simulink model "FDScanningTool2022b"  (R2022b)
settings: Solver=ode1  StartTime=0.0  StopTime=Tobs  FixedStep=delta_t  RelTol=1e-3
values from neighbouring files (symbols this model uses):
  delta_t = 25E-6    (= 2.5e-05)    [exe_FDScanning.m]    (also in exe_FDScanningTool.m = 1e-05)
  dist_time = dist_time_f    [FDScanning.m]    (also in exe_FDScanningTool.m = 1)
  dist_value_0 = Vsignal_dist3    [FDScanning.m]    (also in exe_FDScanningTool.m = 0.05)
  dist_value_a = [Isignal_dist3(:,1),zeros(samples_window,1)]    [FDScanning.m]    (also in exe_FDScanningTool.m)
  dist_value_b = [Isignal_dist3(:,1),zeros(samples_window,1)]    [FDScanning.m]    (also in exe_FDScanningTool.m)
  dist_value_c = Isignal_dist3    [FDScanning.m]    (also in exe_FDScanningTool.m)
  dist_value_d = Isignal_dist1    [FDScanning.m]    (also in exe_FDScanningTool.m = 0.05)
  dist_value_n = [Vsignal_dist3(:,1),zeros(samples_window,1)]    [FDScanning.m]    (also in exe_FDScanningTool.m = 0)
  dist_value_p = [Vsignal_dist3(:,1),zeros(samples_window,1)]    [FDScanning.m]    (also in exe_FDScanningTool.m = 0)
  dist_value_q = [Isignal_dist1(:,1),zeros(samples_window,1)]    [FDScanning.m]    (also in exe_FDScanningTool.m = 0)
  f0 = fs/Ns    [FDScanning.m]    (also in exe_FDScanning.m = 50; exe_FDScanningTool.m = 50)
  fd = fd0(n)    [FDScanning.m]    (also in exe_FDScanningTool.m)
  Id_ss = 0    [exe_FDScanning.m]
  Ipeak = Sbase/Vpeak    [exe_FDScanning.m]    (also in exe_FDScanningTool.m = 1)
  Iq_ss = 0    [exe_FDScanning.m]
  Iss_type = 2    [FDScanning.m]
  phi = (2/3)*pi    (= 2.09439510239)    [FDScanning.m]    (also in exe_FDScanningTool.m)
  Rsource = 1E-6    (= 1e-06)    [FDScanning.m]    (also in exe_FDScanningTool.m = 0.001)
  signal_type = 3    [exe_FDScanning.m]    (also in exe_FDScanningTool.m = 1)
  Vd_ss = 0    [exe_FDScanning.m]
  Vpeak = (Vbase/sqrt(3))*sqrt(2)    [exe_FDScanning.m]    (also in exe_FDScanningTool.m = 1)
  Vq_ss = 0    [exe_FDScanning.m]
  Vss_type = 2    [FDScanning.m]
libraries: spsControlledCurrentSourceLib x12, spsControlledVoltageSourceLib x12, spsThreePhaseVIMeasurementLib x10, spsGroundLib x2, spsThreePhaseSeriesRLCBranchLib x2, spspowerguiLib x1
(part 1 of 2)
settings Model: SimulationMode=accelerator  Creator=Luis Angel  LastModifiedBy=GARREYLU

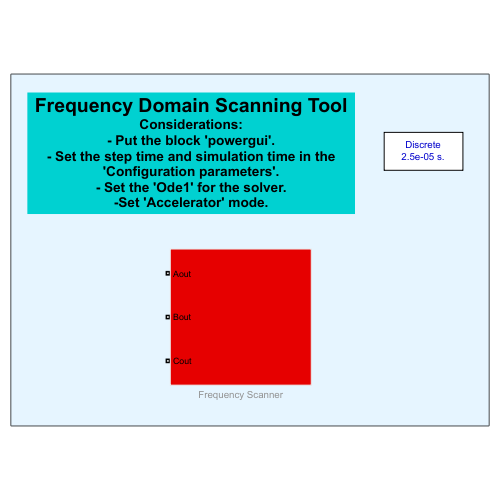
[thumbnail: Simulink's stored preview of the top-level diagram]
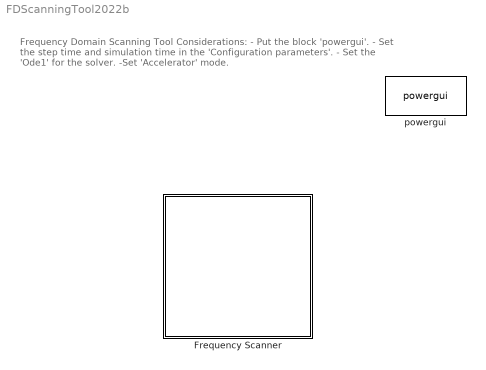
== system FDScanningTool2022b ==
  note: Frequency Domain Scanning Tool
      | Considerations:
      | - Put the block 'powergui'.
      | - Set the step time and simulation time in the 'Configuration parameters'.
      | - Set the 'Ode1' for the solver.
      | -Set 'Accelerator' mode.
  Frequency Scanner : Subsystem
  powergui : spspowerguiLib/powergui  Priority=1  SimulationMode=Discrete  SampleTime=delta_t  frequency=60  Iterations=50  frequencyindice=0  Pbase=100e6  ErrMax=1e-4  UnitsV=kV  UnitsW=MW  buscounter=0  FunctionMessages=off  echomessages=off  EnableUseOfTLC=off  CurrentSourceSwitches=off  DisableSnubberDevices=off  DisableRonSwitches=off  DisableVfSwitches=off  DisplayEquations=off  AutomaticDiscreteSolvers=off  SolverType=Tustin/Backward Euler (TBE)  Interpol=off  ExternalGateDelay=off  methode=off  Ts=100  x0status=blocks  SPID=on  SwTol=0  HookPort=off  NonlinearTolerance=1e-4  nMaxIteration=100  ContinueOnMaxIteration=off  RestoreLinks=warning  ResistiveCurrentMeasurement=off  Frange=[0:2:500]  Ylog=off  Xlog=on  ShowGrid=off  save=off  variable=ZData  structure=0  ZoomFFT=off  StartTime=0.0  cycles=1  DisplayStyle=1  fundamental=60  FreqAxis=off  MaxFrequency=1000  frequencyindicesteady=1  RmsSteady=1  display=off

== system FDScanningTool2022b/Frequency Scanner ==
  note: Current perturbation method
  note: Voltage perturbation method
  Current Strategy : Subsystem  Commented=on
  Three-Phase V-I Measurement1 : spsThreePhaseVIMeasurementLib/Three-Phase V-I Measurement  VoltageMeasurement=no  SetLabelV=on  LabelV=Vabc  Vpu=off  VpuLL=off  CurrentMeasurement=no  SetLabelI=on  LabelI=Iabc  Ipu=off  Pbase=100e6  Vbase=500e3  OutputType=Complex  PhasorSimulation=off  PSBequivalent=0
  Three-Phase V-I Measurement3 : spsThreePhaseVIMeasurementLib/Three-Phase V-I Measurement  VoltageMeasurement=no  SetLabelV=on  LabelV=Vabc  Vpu=off  VpuLL=off  CurrentMeasurement=no  SetLabelI=on  LabelI=Iabc  Ipu=off  Pbase=100e6  Vbase=500e3  OutputType=Complex  PhasorSimulation=off  PSBequivalent=0
  Voltage Strategy : Subsystem
  Aout : PMIOPort  Side=Right
  Bout : PMIOPort  Port=2  Side=Right
  Cout : PMIOPort  Port=3  Side=Right
  connections:
  Bout/RConn1 -- Three-Phase V-I Measurement3/RConn2 -- Three-Phase V-I Measurement1/RConn2
  Aout/RConn1 -- Three-Phase V-I Measurement3/RConn1 -- Three-Phase V-I Measurement1/RConn1
  Cout/RConn1 -- Three-Phase V-I Measurement1/RConn3 -- Three-Phase V-I Measurement3/RConn3
  Three-Phase V-I Measurement1/LConn1 -- Voltage Strategy/RConn1
  Three-Phase V-I Measurement1/LConn2 -- Voltage Strategy/RConn2
  Three-Phase V-I Measurement1/LConn3 -- Voltage Strategy/RConn3
  Three-Phase V-I Measurement3/LConn1 -- Current Strategy/LConn1
  Three-Phase V-I Measurement3/LConn2 -- Current Strategy/LConn2
  Three-Phase V-I Measurement3/LConn3 -- Current Strategy/LConn3

== system FDScanningTool2022b/Frequency Scanner/Current Strategy ==
  note: qd0 scan
  note: Fundamental source
  note: pn0 scan
  note: ABC scan
  ABCdisturbance2 : Subsystem  Commented=on
  Current Fundamental Source : Subsystem
      settings: PortSchema="{\"entries\":[{\"content\":{\"sides\":[{\"content\":{\"connectorIds\":[\"Out1\"]},\"type\":\"ConnectorPlacement.EquallySpacedRectSide\",\"uuid\":\"2a4baa29-0316-4256-b4e1-e3ef1d370b3b\"},{\"content\":{\"connectorIds\":[\"RConn1\",\"RConn2\",\"RConn3\"],\"side\":\"RIGHT\"},\"type\":\"ConnectorPlacement.EquallySpacedRectSide\",\"uuid\":\"3108b85a-ac52-49ed-83a6-d77923640585\"},{\"content\":{\"connectorIds\":[],\"side\":\"TOP\"},\"type\":\"ConnectorPlacement.EquallySpacedRectSide\",\"uuid\":\"4093502e-3b8b-4232-aa57-5a461ca3ca63\"},{\"content\":{\"connectorIds\":[\"RConn4\"],\"side\":\"BOTTOM\"},\"type\":\"ConnectorPlacement.EquallySpacedRectSide\",\"uuid\":\"50c06102-7582-4746-a571-3f791f943454\"}]},\"type\":\"ConnectorPlacement.EquallySpacedConnector\",\"uuid\":\"209f4db4-fe77-48a5-84ae-6773984a343b\"}],\"packageUris\":[\"http://schema.mathworks.com/mf0/Connector/R2020b\"],\"version\":\"1.0\"}"
  Three-Phase V-I Measurement2 : spsThreePhaseVIMeasurementLib/Three-Phase V-I Measurement  VoltageMeasurement=no  SetLabelV=on  LabelV=Vabc  Vpu=off  VpuLL=off  CurrentMeasurement=no  SetLabelI=on  LabelI=Iabc  Ipu=off  Pbase=100e6  Vbase=500e3  OutputType=Complex  PhasorSimulation=off  PSBequivalent=0
  pn0disturbance2 : Subsystem  Commented=on
  qd0disturbance2 : Subsystem
      settings: PortSchema="{\"entries\":[{\"content\":{\"sides\":[{\"content\":{\"connectorIds\":[\"LConn1\",\"LConn2\",\"LConn3\",\"LConn4\"]},\"type\":\"ConnectorPlacement.EquallySpacedRectSide\",\"uuid\":\"96b61a08-e73c-4bf9-b44c-8e6d57b8ef4a\"},{\"content\":{\"connectorIds\":[\"RConn1\",\"RConn2\",\"RConn3\"],\"side\":\"RIGHT\"},\"type\":\"ConnectorPlacement.EquallySpacedRectSide\",\"uuid\":\"3a0e4222-9b60-4a58-9d08-3b159ebff1b9\"},{\"content\":{\"connectorIds\":[\"In1\"],\"side\":\"TOP\"},\"type\":\"ConnectorPlacement.EquallySpacedRectSide\",\"uuid\":\"61af63da-f353-4270-b8c9-89c35459604e\"}]},\"type\":\"ConnectorPlacement.EquallySpacedConnector\",\"uuid\":\"24d596f4-e3d4-42a2-b524-8b1140a91bdb\"}],\"packageUris\":[\"http://schema.mathworks.com/mf0/Connector/R2020b\"],\"version\":\"1.0\"}"
  Aout : PMIOPort  Side=Left
  Bout : PMIOPort  Port=2  Side=Left
  Cout : PMIOPort  Port=3  Side=Left
  wires:
  [theta] -> qd0disturbance2/1(theta)
  Current Fundamental Source/1(theta) -> [theta]
  connections:
  pn0disturbance2/RConn1 -- Aout/RConn1 -- ABCdisturbance2/RConn1 -- qd0disturbance2/RConn1
  pn0disturbance2/RConn2 -- Bout/RConn1 -- ABCdisturbance2/RConn2 -- qd0disturbance2/RConn2
  Current Fundamental Source/RConn2 -- Three-Phase V-I Measurement2/LConn2
  Three-Phase V-I Measurement2/RConn2 -- pn0disturbance2/LConn2 -- ABCdisturbance2/LConn2 -- qd0disturbance2/LConn2
  Current Fundamental Source/RConn3 -- Three-Phase V-I Measurement2/LConn3
  pn0disturbance2/RConn3 -- Cout/RConn1 -- ABCdisturbance2/RConn3 -- qd0disturbance2/RConn3
  Three-Phase V-I Measurement2/RConn1 -- pn0disturbance2/LConn1 -- ABCdisturbance2/LConn1 -- qd0disturbance2/LConn1
  Current Fundamental Source/RConn4 -- pn0disturbance2/LConn4 -- ABCdisturbance2/LConn4 -- qd0disturbance2/LConn4
  Three-Phase V-I Measurement2/RConn3 -- pn0disturbance2/LConn3 -- ABCdisturbance2/LConn3 -- qd0disturbance2/LConn3
  Current Fundamental Source/RConn1 -- Three-Phase V-I Measurement2/LConn1

== system FDScanningTool2022b/Frequency Scanner/Voltage Strategy ==
  note: Fundamental source
  note: pn0 scan
  note: ABC scan
  note: qd0 scan
  ABCdisturbance : Subsystem  Commented=on
  Three-Phase V-I Measurement : spsThreePhaseVIMeasurementLib/Three-Phase V-I Measurement  VoltageMeasurement=no  SetLabelV=on  LabelV=Vabc  Vpu=off  VpuLL=off  CurrentMeasurement=no  SetLabelI=on  LabelI=Iabc  Ipu=off  Pbase=100e6  Vbase=500e3  OutputType=Complex  PhasorSimulation=off  PSBequivalent=0
  Voltage Fundamental Source : Subsystem
      settings: PortSchema="{\"entries\":[{\"content\":{\"sides\":[{\"content\":{\"connectorIds\":[\"Out1\"]},\"type\":\"ConnectorPlacement.EquallySpacedRectSide\",\"uuid\":\"3dbf8d23-22ab-4ddc-ae4a-19197e180312\"},{\"content\":{\"connectorIds\":[\"RConn1\",\"RConn2\",\"RConn3\"],\"side\":\"RIGHT\"},\"type\":\"ConnectorPlacement.EquallySpacedRectSide\",\"uuid\":\"df914263-db35-4888-aa99-5dec7a54c6e0\"},{\"content\":{\"connectorIds\":[],\"side\":\"TOP\"},\"type\":\"ConnectorPlacement.EquallySpacedRectSide\",\"uuid\":\"815bd59d-9d4f-4637-8c0a-95368e7d07f9\"}]},\"type\":\"ConnectorPlacement.EquallySpacedConnector\",\"uuid\":\"b7ffca83-a6f6-4340-8cfa-6aec16cec0d1\"}],\"packageUris\":[\"http://schema.mathworks.com/mf0/Connector/R2020b\"],\"version\":\"1.0\"}"
  pn0disturbance : Subsystem  Commented=on
  qd0disturbance : Subsystem
      settings: PortSchema="{\"entries\":[{\"content\":{\"sides\":[{\"content\":{\"connectorIds\":[\"LConn1\",\"LConn2\",\"LConn3\"]},\"type\":\"ConnectorPlacement.EquallySpacedRectSide\",\"uuid\":\"96b61a08-e73c-4bf9-b44c-8e6d57b8ef4a\"},{\"content\":{\"connectorIds\":[\"RConn1\",\"RConn2\",\"RConn3\"],\"side\":\"RIGHT\"},\"type\":\"ConnectorPlacement.EquallySpacedRectSide\",\"uuid\":\"3a0e4222-9b60-4a58-9d08-3b159ebff1b9\"},{\"content\":{\"connectorIds\":[\"In1\"],\"side\":\"TOP\"},\"type\":\"ConnectorPlacement.EquallySpacedRectSide\",\"uuid\":\"61af63da-f353-4270-b8c9-89c35459604e\"}]},\"type\":\"ConnectorPlacement.EquallySpacedConnector\",\"uuid\":\"24d596f4-e3d4-42a2-b524-8b1140a91bdb\"}],\"packageUris\":[\"http://schema.mathworks.com/mf0/Connector/R2020b\"],\"version\":\"1.0\"}"
  Aout : PMIOPort  Side=Right
  Bout : PMIOPort  Port=2  Side=Right
  Cout : PMIOPort  Port=3  Side=Right
  wires:
  Voltage Fundamental Source/1(theta) -> [theta]
  [theta] -> qd0disturbance/1(theta)
  connections:
  ABCdisturbance/RConn2 -- Bout/RConn1 -- pn0disturbance/RConn2 -- qd0disturbance/RConn2
  Voltage Fundamental Source/RConn1 -- Three-Phase V-I Measurement/LConn1
  qd0disturbance/LConn3 -- ABCdisturbance/LConn3 -- Three-Phase V-I Measurement/RConn3 -- pn0disturbance/LConn3
  ABCdisturbance/RConn1 -- Aout/RConn1 -- pn0disturbance/RConn1 -- qd0disturbance/RConn1
  Voltage Fundamental Source/RConn2 -- Three-Phase V-I Measurement/LConn2
  Voltage Fundamental Source/RConn3 -- Three-Phase V-I Measurement/LConn3
  ABCdisturbance/RConn3 -- Cout/RConn1 -- pn0disturbance/RConn3 -- qd0disturbance/RConn3
  qd0disturbance/LConn1 -- ABCdisturbance/LConn1 -- Three-Phase V-I Measurement/RConn1 -- pn0disturbance/LConn1
  qd0disturbance/LConn2 -- ABCdisturbance/LConn2 -- Three-Phase V-I Measurement/RConn2 -- pn0disturbance/LConn2

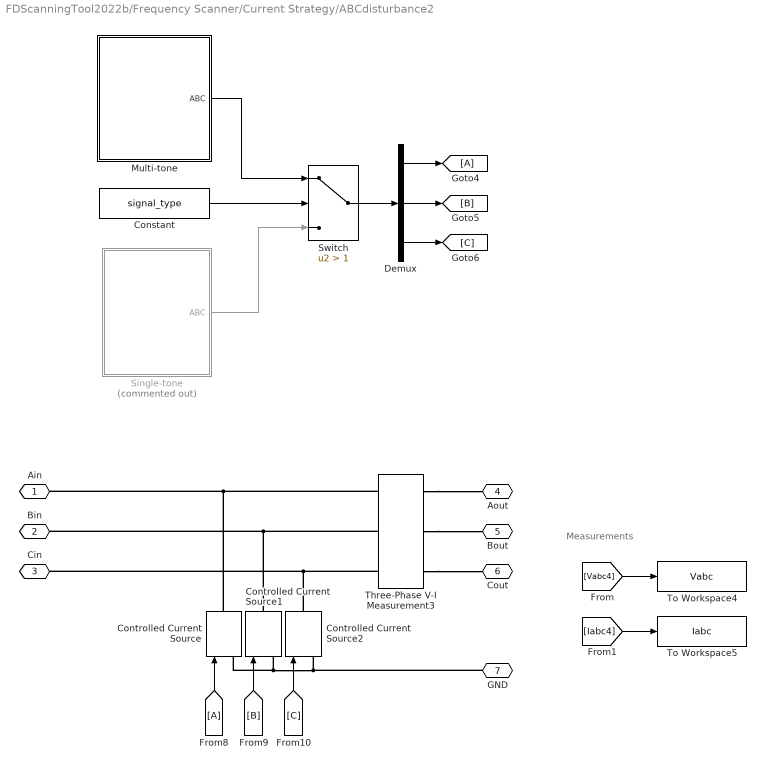
== system FDScanningTool2022b/Frequency Scanner/Current Strategy/ABCdisturbance2 ==
  note: Measurements
  Constant : Constant  Value=signal_type
  Controlled Current Source : spsControlledCurrentSourceLib/Controlled Current Source  Initialize=off  Source_Type=AC  Amplitude=0  Phase=0  Frequency=0  Measurements=None
  Controlled Current Source1 : spsControlledCurrentSourceLib/Controlled Current Source  Initialize=off  Source_Type=AC  Amplitude=0  Phase=0  Frequency=0  Measurements=None
  Controlled Current Source2 : spsControlledCurrentSourceLib/Controlled Current Source  Initialize=off  Source_Type=AC  Amplitude=0  Phase=0  Frequency=0  Measurements=None
  Demux : Demux  Outputs=3
  From8 : From
  Goto4 : Goto
  Multi-tone : Subsystem
  Single-tone : Subsystem  Commented=on
  Switch : Switch  Criteria=u2 > Threshold  Threshold=1  SaturateOnIntegerOverflow=off  InputSameDT=off
  Three-Phase V-I Measurement3 : spsThreePhaseVIMeasurementLib/Three-Phase V-I Measurement  VoltageMeasurement=phase-to-ground  SetLabelV=on  LabelV=Vabc4  Vpu=off  VpuLL=off  CurrentMeasurement=yes  SetLabelI=on  LabelI=Iabc4  Ipu=off  Pbase=100e6  Vbase=500e3  OutputType=Complex  PhasorSimulation=off  PSBequivalent=0
  To Workspace4 : ToWorkspace  VariableName=Vabc  SampleTime=-1
  To Workspace5 : ToWorkspace  VariableName=Iabc  SampleTime=-1
  Ain : PMIOPort  Side=Left
  Bin : PMIOPort  Port=2  Side=Left
  Cin : PMIOPort  Port=3  Side=Left
  Aout : PMIOPort  Port=4  Side=Right
  Bout : PMIOPort  Port=5  Side=Right
  Cout : PMIOPort  Port=6  Side=Right
  GND : PMIOPort  Port=7  Side=Left
  wires:
  [Vabc4] -> To Workspace4/1
  [Iabc4] -> To Workspace5/1
  [C] -> Controlled Current Source2/1
  [B] -> Controlled Current Source1/1
  From8/1 -> Controlled Current Source/1
  Constant/1 -> Switch/2
  Multi-tone/1(ABC) -> Switch/1
  Demux/1 -> Goto4/1
  Demux/2 -> [B]
  Demux/3 -> [C]
  Switch/1 -> Demux/1
  Single-tone/1(ABC) -> Switch/3
  connections:
  Controlled Current Source1/LConn1 -- GND/RConn1 -- Controlled Current Source2/LConn1 -- Controlled Current Source/LConn1
  Controlled Current Source/RConn1 -- Three-Phase V-I Measurement3/LConn1 -- Ain/RConn1
  Controlled Current Source2/RConn1 -- Three-Phase V-I Measurement3/LConn3 -- Cin/RConn1
  Controlled Current Source1/RConn1 -- Three-Phase V-I Measurement3/LConn2 -- Bin/RConn1
  Three-Phase V-I Measurement3/RConn1 -- Aout/RConn1
  Three-Phase V-I Measurement3/RConn2 -- Bout/RConn1
  Three-Phase V-I Measurement3/RConn3 -- Cout/RConn1

== system FDScanningTool2022b/Frequency Scanner/Current Strategy/Current Fundamental Source ==
  Controlled Current Source : spsControlledCurrentSourceLib/Controlled Current Source  Initialize=off  Source_Type=AC  Amplitude=0  Phase=0  Frequency=0  Measurements=None
  Controlled Current Source1 : spsControlledCurrentSourceLib/Controlled Current Source  Initialize=off  Source_Type=AC  Amplitude=0  Phase=0  Frequency=0  Measurements=None
  Controlled Current Source2 : spsControlledCurrentSourceLib/Controlled Current Source  Initialize=off  Source_Type=AC  Amplitude=0  Phase=0  Frequency=0  Measurements=None
  Grid Currents1 : Subsystem
  Ground : spsGroundLib/Ground  LConnTagsString=a
  Three-Phase Series RLC Branch : spsThreePhaseSeriesRLCBranchLib/Three-Phase Series RLC Branch  LConnTagsString=A|B|C  RConnTagsString=A|B|C  BranchType=R  Resistance=1/Rsource  Inductance=1e-3  Capacitance=1e-6  Measurements=None
  VzA : PMIOPort  Side=Right
  VzB : PMIOPort  Port=2  Side=Right
  VzC : PMIOPort  Port=3  Side=Right
  GND : PMIOPort  Port=4  Side=Right
  theta : Outport
  wires:
  Grid Currents1/3(IC) -> Controlled Current Source/1
  Grid Currents1/2(IB) -> Controlled Current Source1/1
  Grid Currents1/1(IA) -> Controlled Current Source2/1
  Grid Currents1/4(theta) -> theta/1
  connections:
  Controlled Current Source2/RConn1 -- Three-Phase Series RLC Branch/LConn1 -- VzA/RConn1
  Controlled Current Source1/RConn1 -- Three-Phase Series RLC Branch/LConn2 -- VzB/RConn1
  Controlled Current Source/RConn1 -- Three-Phase Series RLC Branch/LConn3 -- VzC/RConn1
  Ground/LConn1 -- Controlled Current Source/LConn1 -- Controlled Current Source1/LConn1 -- Controlled Current Source2/LConn1 -- Three-Phase Series RLC Branch/RConn3 -- Three-Phase Series RLC Branch/RConn2 -- Three-Phase Series RLC Branch/RConn1 -- GND/RConn1

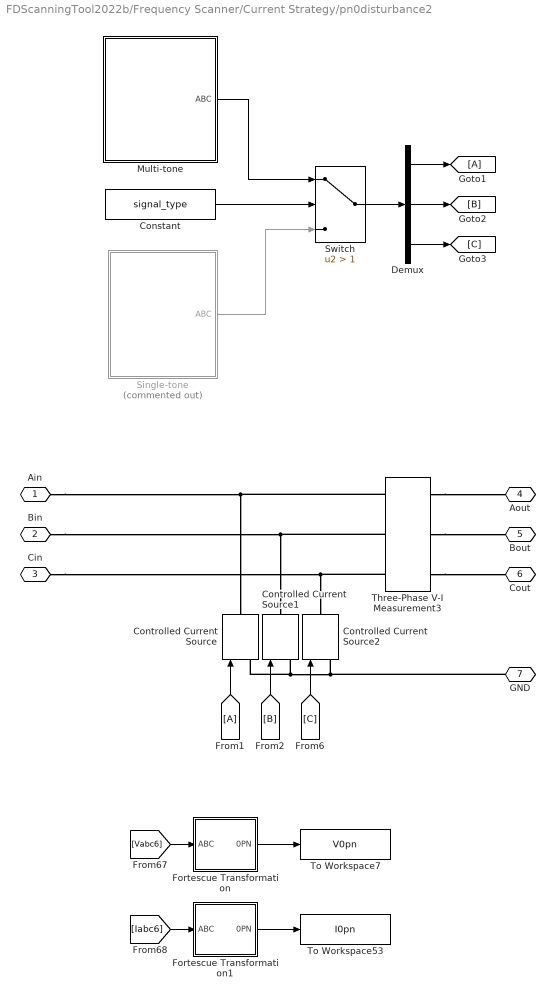
== system FDScanningTool2022b/Frequency Scanner/Current Strategy/pn0disturbance2 ==
  Constant : Constant  Value=signal_type
  Controlled Current Source : spsControlledCurrentSourceLib/Controlled Current Source  Initialize=off  Source_Type=AC  Amplitude=0  Phase=0  Frequency=0  Measurements=None
  Controlled Current Source1 : spsControlledCurrentSourceLib/Controlled Current Source  Initialize=off  Source_Type=AC  Amplitude=0  Phase=0  Frequency=0  Measurements=None
  Controlled Current Source2 : spsControlledCurrentSourceLib/Controlled Current Source  Initialize=off  Source_Type=AC  Amplitude=0  Phase=0  Frequency=0  Measurements=None
  Demux : Demux  Outputs=3
  Fortescue Transformation : Subsystem
  Fortescue Transformation1 : Subsystem
  From1 : From
  Goto1 : Goto
  Multi-tone : Subsystem
  Single-tone : Subsystem  Commented=on
  Switch : Switch  Criteria=u2 > Threshold  Threshold=1  SaturateOnIntegerOverflow=off  InputSameDT=off
  Three-Phase V-I Measurement3 : spsThreePhaseVIMeasurementLib/Three-Phase V-I Measurement  VoltageMeasurement=phase-to-ground  SetLabelV=on  LabelV=Vabc6  Vpu=off  VpuLL=off  CurrentMeasurement=yes  SetLabelI=on  LabelI=Iabc6  Ipu=off  Pbase=100e6  Vbase=500e3  OutputType=Complex  PhasorSimulation=off  PSBequivalent=0
  To Workspace53 : ToWorkspace  VariableName=I0pn  SampleTime=-1
  To Workspace7 : ToWorkspace  VariableName=V0pn  SampleTime=-1
  Ain : PMIOPort  Side=Left
  Bin : PMIOPort  Port=2  Side=Left
  Cin : PMIOPort  Port=3  Side=Left
  Aout : PMIOPort  Port=4  Side=Right
  Bout : PMIOPort  Port=5  Side=Right
  Cout : PMIOPort  Port=6  Side=Right
  GND : PMIOPort  Port=7  Side=Left
  wires:
  [Vabc6] -> Fortescue Transformation/1(ABC)
  [Iabc6] -> Fortescue Transformation1/1(ABC)
  Fortescue Transformation/1(0PN) -> To Workspace7/1
  Fortescue Transformation1/1(0PN) -> To Workspace53/1
  [B] -> Controlled Current Source1/1
  [C] -> Controlled Current Source2/1
  From1/1 -> Controlled Current Source/1
  Multi-tone/1(ABC) -> Switch/1
  Demux/1 -> Goto1/1
  Demux/3 -> [C]
  Constant/1 -> Switch/2
  Single-tone/1(ABC) -> Switch/3
  Switch/1 -> Demux/1
  Demux/2 -> [B]
  connections:
  Cin/RConn1 -- Three-Phase V-I Measurement3/LConn3 -- Controlled Current Source2/RConn1
  Controlled Current Source1/LConn1 -- GND/RConn1 -- Controlled Current Source2/LConn1 -- Controlled Current Source/LConn1
  Ain/RConn1 -- Three-Phase V-I Measurement3/LConn1 -- Controlled Current Source/RConn1
  Bin/RConn1 -- Three-Phase V-I Measurement3/LConn2 -- Controlled Current Source1/RConn1
  Three-Phase V-I Measurement3/RConn3 -- Cout/RConn1
  Three-Phase V-I Measurement3/RConn2 -- Bout/RConn1
  Three-Phase V-I Measurement3/RConn1 -- Aout/RConn1

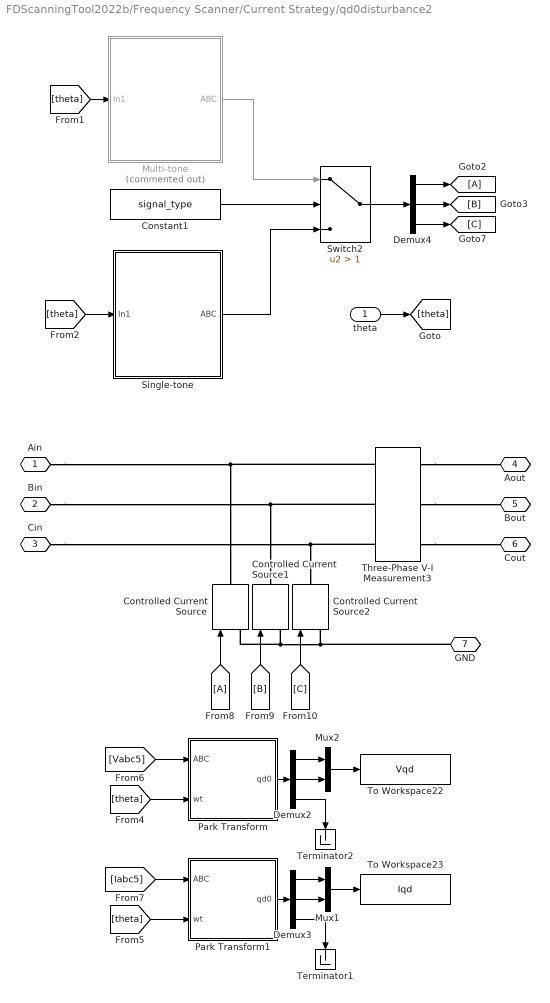
== system FDScanningTool2022b/Frequency Scanner/Current Strategy/qd0disturbance2 ==
  theta : Inport
  Constant1 : Constant  Value=signal_type
  Controlled Current Source : spsControlledCurrentSourceLib/Controlled Current Source  Initialize=off  Source_Type=AC  Amplitude=0  Phase=0  Frequency=0  Measurements=None
  Controlled Current Source1 : spsControlledCurrentSourceLib/Controlled Current Source  Initialize=off  Source_Type=AC  Amplitude=0  Phase=0  Frequency=0  Measurements=None
  Controlled Current Source2 : spsControlledCurrentSourceLib/Controlled Current Source  Initialize=off  Source_Type=AC  Amplitude=0  Phase=0  Frequency=0  Measurements=None
  Demux2 : Demux  Outputs=3
  Demux3 : Demux  Outputs=3
  Demux4 : Demux  Outputs=3
  From8 : From
  Goto2 : Goto
  Multi-tone : Subsystem  Commented=on
  Mux1 : Mux  Inputs=2
  Mux2 : Mux  Inputs=2
  Park Transform : Subsystem
  Park Transform1 : Subsystem
  Single-tone : Subsystem
  Switch2 : Switch  Criteria=u2 > Threshold  Threshold=1  SaturateOnIntegerOverflow=off  InputSameDT=off
  Terminator1 : Terminator
  Terminator2 : Terminator
  Three-Phase V-I Measurement3 : spsThreePhaseVIMeasurementLib/Three-Phase V-I Measurement  VoltageMeasurement=phase-to-ground  SetLabelV=on  LabelV=Vabc5  Vpu=off  VpuLL=off  CurrentMeasurement=yes  SetLabelI=on  LabelI=Iabc5  Ipu=off  Pbase=100e6  Vbase=500e3  OutputType=Complex  PhasorSimulation=off  PSBequivalent=0
  To Workspace22 : ToWorkspace  VariableName=Vqd  SampleTime=-1
  To Workspace23 : ToWorkspace  VariableName=Iqd  SampleTime=-1
  Ain : PMIOPort  Side=Left
  Bin : PMIOPort  Port=2  Side=Left
  Cin : PMIOPort  Port=3  Side=Left
  Aout : PMIOPort  Port=4  Side=Right
  Bout : PMIOPort  Port=5  Side=Right
  Cout : PMIOPort  Port=6  Side=Right
  GND : PMIOPort  Port=7  Side=Left
  wires:
  Mux2/1 -> To Workspace22/1
  [theta] -> Park Transform/2(wt)
  [Vabc5] -> Park Transform/1(ABC)
  Park Transform/1(qd0) -> Demux2/1
  Demux2/3 -> Terminator2/1
  theta/1 -> [theta]
  Demux2/1 -> Mux2/1
  Demux2/2 -> Mux2/2
  Mux1/1 -> To Workspace23/1
  Demux3/3 -> Terminator1/1
  [Iabc5] -> Park Transform1/1(ABC)
  Park Transform1/1(qd0) -> Demux3/1
  Demux3/2 -> Mux1/2
  Demux3/1 -> Mux1/1
  [theta] -> Park Transform1/2(wt)
  From8/1 -> Controlled Current Source/1
  [C] -> Controlled Current Source2/1
  [B] -> Controlled Current Source1/1
  Constant1/1 -> Switch2/2
  Multi-tone/1(ABC) -> Switch2/1
  [theta] -> Single-tone/1(In1)
  Switch2/1 -> Demux4/1
  Single-tone/1(ABC) -> Switch2/3
  Demux4/1 -> Goto2/1
  Demux4/2 -> [B]
  [theta] -> Multi-tone/1(In1)
  Demux4/3 -> [C]
  connections:
  Controlled Current Source1/LConn1 -- GND/RConn1 -- Controlled Current Source2/LConn1 -- Controlled Current Source/LConn1
  Ain/RConn1 -- Three-Phase V-I Measurement3/LConn1 -- Controlled Current Source/RConn1
  Bin/RConn1 -- Three-Phase V-I Measurement3/LConn2 -- Controlled Current Source1/RConn1
  Cin/RConn1 -- Three-Phase V-I Measurement3/LConn3 -- Controlled Current Source2/RConn1
  Three-Phase V-I Measurement3/RConn1 -- Aout/RConn1
  Three-Phase V-I Measurement3/RConn2 -- Bout/RConn1
  Three-Phase V-I Measurement3/RConn3 -- Cout/RConn1

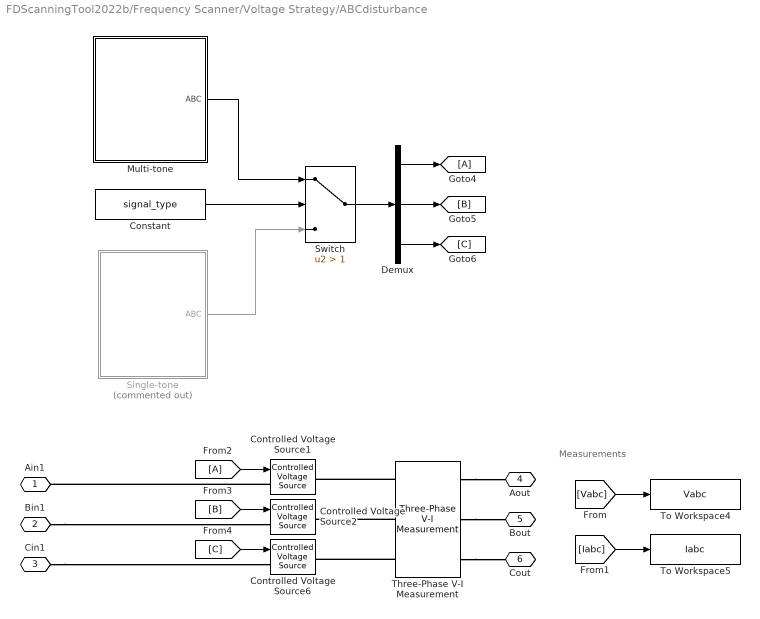
== system FDScanningTool2022b/Frequency Scanner/Voltage Strategy/ABCdisturbance ==
  note: Measurements
  Constant : Constant  Value=signal_type
  Controlled Voltage Source1 : spsControlledVoltageSourceLib/Controlled Voltage Source  Initialize=off  Source_Type=DC  Amplitude=0  Phase=0  Frequency=0  Measurements=None
  Controlled Voltage Source2 : spsControlledVoltageSourceLib/Controlled Voltage Source  Initialize=off  Source_Type=DC  Amplitude=0  Phase=0  Frequency=0  Measurements=None
  Controlled Voltage Source6 : spsControlledVoltageSourceLib/Controlled Voltage Source  Initialize=off  Source_Type=DC  Amplitude=0  Phase=0  Frequency=0  Measurements=None
  Demux : Demux  Outputs=3
  From2 : From
  Goto4 : Goto
  Multi-tone : Subsystem
  Single-tone : Subsystem  Commented=on
  Switch : Switch  Criteria=u2 > Threshold  Threshold=1  SaturateOnIntegerOverflow=off  InputSameDT=off
  Three-Phase V-I Measurement : spsThreePhaseVIMeasurementLib/Three-Phase V-I Measurement  VoltageMeasurement=phase-to-ground  SetLabelV=on  LabelV=Vabc  Vpu=off  VpuLL=off  CurrentMeasurement=yes  SetLabelI=on  LabelI=Iabc  Ipu=off  Pbase=100e6  Vbase=500e3  OutputType=Complex  PhasorSimulation=off  PSBequivalent=0
  To Workspace4 : ToWorkspace  VariableName=Vabc  SampleTime=-1
  To Workspace5 : ToWorkspace  VariableName=Iabc  SampleTime=-1
  Ain1 : PMIOPort  Side=Left
  Bin1 : PMIOPort  Port=2  Side=Left
  Cin1 : PMIOPort  Port=3  Side=Left
  Aout : PMIOPort  Port=4  Side=Right
  Bout : PMIOPort  Port=5  Side=Right
  Cout : PMIOPort  Port=6  Side=Right
  wires:
  [Vabc] -> To Workspace4/1
  [Iabc] -> To Workspace5/1
  [C] -> Controlled Voltage Source6/1
  From2/1 -> Controlled Voltage Source1/1
  [B] -> Controlled Voltage Source2/1
  Multi-tone/1(ABC) -> Switch/1
  Demux/3 -> [C]
  Constant/1 -> Switch/2
  Demux/1 -> Goto4/1
  Demux/2 -> [B]
  Single-tone/1(ABC) -> Switch/3
  Switch/1 -> Demux/1
  connections:
  Bin1/RConn1 -- Controlled Voltage Source2/LConn1
  Controlled Voltage Source1/LConn1 -- Ain1/RConn1
  Cin1/RConn1 -- Controlled Voltage Source6/LConn1
  Three-Phase V-I Measurement/LConn1 -- Controlled Voltage Source1/RConn1
  Three-Phase V-I Measurement/LConn2 -- Controlled Voltage Source2/RConn1
  Three-Phase V-I Measurement/LConn3 -- Controlled Voltage Source6/RConn1
  Three-Phase V-I Measurement/RConn3 -- Cout/RConn1
  Three-Phase V-I Measurement/RConn2 -- Bout/RConn1
  Three-Phase V-I Measurement/RConn1 -- Aout/RConn1

== system FDScanningTool2022b/Frequency Scanner/Voltage Strategy/Voltage Fundamental Source ==
  Controlled Voltage Source1 : spsControlledVoltageSourceLib/Controlled Voltage Source  Initialize=off  Source_Type=DC  Amplitude=0  Phase=0  Frequency=0  Measurements=None
  Controlled Voltage Source2 : spsControlledVoltageSourceLib/Controlled Voltage Source  Initialize=off  Source_Type=DC  Amplitude=0  Phase=0  Frequency=0  Measurements=None
  Controlled Voltage Source3 : spsControlledVoltageSourceLib/Controlled Voltage Source  Initialize=off  Source_Type=DC  Amplitude=0  Phase=0  Frequency=0  Measurements=None
  Grid Voltages : Subsystem
  Ground : spsGroundLib/Ground  LConnTagsString=a
  Three-Phase Series RLC Branch : spsThreePhaseSeriesRLCBranchLib/Three-Phase Series RLC Branch  LConnTagsString=A|B|C  RConnTagsString=A|B|C  BranchType=R  Resistance=Rsource  Inductance=1e-3  Capacitance=1e-6  Measurements=None
  VzA : PMIOPort  Side=Right
  VzB : PMIOPort  Port=2  Side=Right
  VzC : PMIOPort  Port=3  Side=Right
  theta : Outport
  wires:
  Grid Voltages/3(VC) -> Controlled Voltage Source3/1
  Grid Voltages/2(VB) -> Controlled Voltage Source2/1
  Grid Voltages/1(VA) -> Controlled Voltage Source1/1
  Grid Voltages/4(theta) -> theta/1
  connections:
  Controlled Voltage Source2/LConn1 -- Controlled Voltage Source1/LConn1 -- Controlled Voltage Source3/LConn1 -- Ground/LConn1
  Three-Phase Series RLC Branch/RConn1 -- Controlled Voltage Source1/RConn1
  Three-Phase Series RLC Branch/RConn2 -- Controlled Voltage Source2/RConn1
  Three-Phase Series RLC Branch/RConn3 -- Controlled Voltage Source3/RConn1
  Three-Phase Series RLC Branch/LConn3 -- VzC/RConn1
  Three-Phase Series RLC Branch/LConn2 -- VzB/RConn1
  Three-Phase Series RLC Branch/LConn1 -- VzA/RConn1

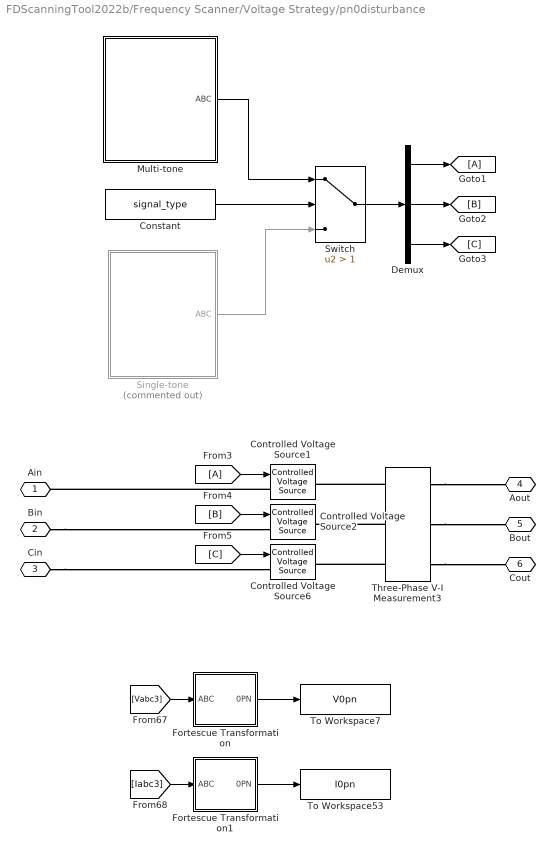
== system FDScanningTool2022b/Frequency Scanner/Voltage Strategy/pn0disturbance ==
  Constant : Constant  Value=signal_type
  Controlled Voltage Source1 : spsControlledVoltageSourceLib/Controlled Voltage Source  Initialize=off  Source_Type=DC  Amplitude=0  Phase=0  Frequency=0  Measurements=None
  Controlled Voltage Source2 : spsControlledVoltageSourceLib/Controlled Voltage Source  Initialize=off  Source_Type=DC  Amplitude=0  Phase=0  Frequency=0  Measurements=None
  Controlled Voltage Source6 : spsControlledVoltageSourceLib/Controlled Voltage Source  Initialize=off  Source_Type=DC  Amplitude=0  Phase=0  Frequency=0  Measurements=None
  Demux : Demux  Outputs=3
  Fortescue Transformation : Subsystem
  Fortescue Transformation1 : Subsystem
  From3 : From
  Goto1 : Goto
  Multi-tone : Subsystem
  Single-tone : Subsystem  Commented=on
  Switch : Switch  Criteria=u2 > Threshold  Threshold=1  SaturateOnIntegerOverflow=off  InputSameDT=off
  Three-Phase V-I Measurement3 : spsThreePhaseVIMeasurementLib/Three-Phase V-I Measurement  VoltageMeasurement=phase-to-ground  SetLabelV=on  LabelV=Vabc3  Vpu=off  VpuLL=off  CurrentMeasurement=yes  SetLabelI=on  LabelI=Iabc3  Ipu=off  Pbase=100e6  Vbase=500e3  OutputType=Complex  PhasorSimulation=off  PSBequivalent=0
  To Workspace53 : ToWorkspace  VariableName=I0pn  SampleTime=-1
  To Workspace7 : ToWorkspace  VariableName=V0pn  SampleTime=-1
  Ain : PMIOPort  Side=Left
  Bin : PMIOPort  Port=2  Side=Left
  Cin : PMIOPort  Port=3  Side=Left
  Aout : PMIOPort  Port=4  Side=Right
  Bout : PMIOPort  Port=5  Side=Right
  Cout : PMIOPort  Port=6  Side=Right
  wires:
  [B] -> Controlled Voltage Source2/1
  From3/1 -> Controlled Voltage Source1/1
  [C] -> Controlled Voltage Source6/1
  [Vabc3] -> Fortescue Transformation/1(ABC)
  [Iabc3] -> Fortescue Transformation1/1(ABC)
  Fortescue Transformation/1(0PN) -> To Workspace7/1
  Fortescue Transformation1/1(0PN) -> To Workspace53/1
  Switch/1 -> Demux/1
  Single-tone/1(ABC) -> Switch/3
  Demux/3 -> [C]
  Multi-tone/1(ABC) -> Switch/1
  Demux/1 -> Goto1/1
  Demux/2 -> [B]
  Constant/1 -> Switch/2
  connections:
  Controlled Voltage Source1/LConn1 -- Ain/RConn1
  Cin/RConn1 -- Controlled Voltage Source6/LConn1
  Bin/RConn1 -- Controlled Voltage Source2/LConn1
  Three-Phase V-I Measurement3/LConn1 -- Controlled Voltage Source1/RConn1
  Three-Phase V-I Measurement3/LConn2 -- Controlled Voltage Source2/RConn1
  Three-Phase V-I Measurement3/LConn3 -- Controlled Voltage Source6/RConn1
  Three-Phase V-I Measurement3/RConn1 -- Aout/RConn1
  Three-Phase V-I Measurement3/RConn2 -- Bout/RConn1
  Three-Phase V-I Measurement3/RConn3 -- Cout/RConn1

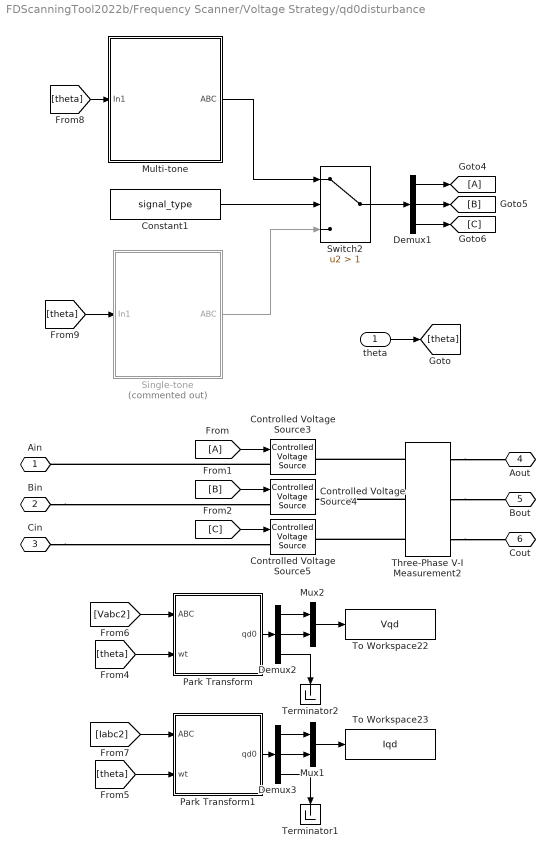
== system FDScanningTool2022b/Frequency Scanner/Voltage Strategy/qd0disturbance ==
  theta : Inport
  Constant1 : Constant  Value=signal_type
  Controlled Voltage Source3 : spsControlledVoltageSourceLib/Controlled Voltage Source  Initialize=off  Source_Type=DC  Amplitude=0  Phase=0  Frequency=0  Measurements=None
  Controlled Voltage Source4 : spsControlledVoltageSourceLib/Controlled Voltage Source  Initialize=off  Source_Type=DC  Amplitude=0  Phase=0  Frequency=0  Measurements=None
  Controlled Voltage Source5 : spsControlledVoltageSourceLib/Controlled Voltage Source  Initialize=off  Source_Type=DC  Amplitude=0  Phase=0  Frequency=0  Measurements=None
  Demux1 : Demux  Outputs=3
  Demux2 : Demux  Outputs=3
  Demux3 : Demux  Outputs=3
  From : From
  Goto4 : Goto
  Multi-tone : Subsystem
  Mux1 : Mux  Inputs=2
  Mux2 : Mux  Inputs=2
  Park Transform : Subsystem
  Park Transform1 : Subsystem
  Single-tone : Subsystem  Commented=on
  Switch2 : Switch  Criteria=u2 > Threshold  Threshold=1  SaturateOnIntegerOverflow=off  InputSameDT=off
  Terminator1 : Terminator
  Terminator2 : Terminator
  Three-Phase V-I Measurement2 : spsThreePhaseVIMeasurementLib/Three-Phase V-I Measurement  VoltageMeasurement=phase-to-ground  SetLabelV=on  LabelV=Vabc2  Vpu=off  VpuLL=off  CurrentMeasurement=yes  SetLabelI=on  LabelI=Iabc2  Ipu=off  Pbase=100e6  Vbase=500e3  OutputType=Complex  PhasorSimulation=off  PSBequivalent=0
  To Workspace22 : ToWorkspace  VariableName=Vqd  SampleTime=-1
  To Workspace23 : ToWorkspace  VariableName=Iqd  SampleTime=-1
  Ain : PMIOPort  Side=Left
  Bin : PMIOPort  Port=2  Side=Left
  Cin : PMIOPort  Port=3  Side=Left
  Aout : PMIOPort  Port=4  Side=Right
  Bout : PMIOPort  Port=5  Side=Right
  Cout : PMIOPort  Port=6  Side=Right
  wires:
  From/1 -> Controlled Voltage Source3/1
  [B] -> Controlled Voltage Source4/1
  [C] -> Controlled Voltage Source5/1
  Mux2/1 -> To Workspace22/1
  [theta] -> Park Transform/2(wt)
  [Vabc2] -> Park Transform/1(ABC)
  Park Transform/1(qd0) -> Demux2/1
  Demux2/3 -> Terminator2/1
  theta/1 -> [theta]
  Demux2/1 -> Mux2/1
  Demux2/2 -> Mux2/2
  Mux1/1 -> To Workspace23/1
  Demux3/3 -> Terminator1/1
  [Iabc2] -> Park Transform1/1(ABC)
  Park Transform1/1(qd0) -> Demux3/1
  Demux3/2 -> Mux1/2
  Demux3/1 -> Mux1/1
  [theta] -> Park Transform1/2(wt)
  Switch2/1 -> Demux1/1
  Single-tone/1(ABC) -> Switch2/3
  Multi-tone/1(ABC) -> Switch2/1
  Constant1/1 -> Switch2/2
  [theta] -> Single-tone/1(In1)
  Demux1/3 -> [C]
  Demux1/1 -> Goto4/1
  Demux1/2 -> [B]
  [theta] -> Multi-tone/1(In1)
  connections:
  Controlled Voltage Source3/LConn1 -- Ain/RConn1
  Bin/RConn1 -- Controlled Voltage Source4/LConn1
  Cin/RConn1 -- Controlled Voltage Source5/LConn1
  Three-Phase V-I Measurement2/LConn1 -- Controlled Voltage Source3/RConn1
  Three-Phase V-I Measurement2/LConn2 -- Controlled Voltage Source4/RConn1
  Three-Phase V-I Measurement2/LConn3 -- Controlled Voltage Source5/RConn1
  Three-Phase V-I Measurement2/RConn1 -- Aout/RConn1
  Three-Phase V-I Measurement2/RConn2 -- Bout/RConn1
  Three-Phase V-I Measurement2/RConn3 -- Cout/RConn1

== system FDScanningTool2022b/Frequency Scanner/Current Strategy/ABCdisturbance2/Multi-tone ==
  Clock : Clock
  Constant1 : Constant  Value=0
  From Workspace : FromWorkspace  VariableName=dist_value_a  SampleTime=delta_t  Interpolate=off  OutputAfterFinalValue=Holding final value
  From Workspace1 : FromWorkspace  VariableName=dist_value_b  SampleTime=delta_t  Interpolate=off  OutputAfterFinalValue=Holding final value
  From Workspace2 : FromWorkspace  VariableName=dist_value_c  SampleTime=delta_t  Interpolate=off  OutputAfterFinalValue=Holding final value
  Mux : Mux  Inputs=3
  Switch1 : Switch  Criteria=u2 > Threshold  Threshold=dist_time  SaturateOnIntegerOverflow=off  InputSameDT=off
  Switch2 : Switch  Criteria=u2 > Threshold  Threshold=dist_time  SaturateOnIntegerOverflow=off  InputSameDT=off
  Switch3 : Switch  Criteria=u2 > Threshold  Threshold=dist_time  SaturateOnIntegerOverflow=off  InputSameDT=off
  ABC : Outport
  wires:
  Switch2/1 -> Mux/2
  From Workspace2/1 -> Switch3/1
  Constant1/1 -> Switch3/3, Switch2/3, Switch1/3
  From Workspace1/1 -> Switch2/1
  Switch3/1 -> Mux/3
  Clock/1 -> Switch1/2, Switch2/2, Switch3/2
  Switch1/1 -> Mux/1
  From Workspace/1 -> Switch1/1
  Mux/1 -> ABC/1

== system FDScanningTool2022b/Frequency Scanner/Current Strategy/ABCdisturbance2/Single-tone ==
  note: ABC perturbance
  Constant10 : Constant  Value=phi
  Constant12 : Constant  Value=2*pi*fd  SampleTime=delta_t
  Constant9 : Constant  Value=phi
  Integrator5 : Integrator  UpperSaturationLimit=1E100  LowerSaturationLimit=-1E100
  Mux : Mux  Inputs=3
  Product1 : Product
  Product2 : Product
  Product3 : Product
  Sin : Trigonometry  Operator=cos
  Sin1 : Trigonometry  Operator=cos
  Sin2 : Trigonometry  Operator=cos
  Step1 : Step  Time=dist_time  After=dist_value_a  SampleTime=delta_t
  Step2 : Step  Time=dist_time  After=dist_value_b  SampleTime=delta_t
  Step3 : Step  Time=dist_time  After=dist_value_c  SampleTime=delta_t
  Sum6 : Sum  Inputs=|+-
  Sum7 : Sum  Inputs=|++
  ABC : Outport
  wires:
  Sin/1 -> Product1/1
  Sum7/1 -> Sin2/1
  Product1/1 -> Mux/1
  Integrator5/1 -> Sum7/1, Sin/1, Sum6/1
  Sin1/1 -> Product2/1
  Sin2/1 -> Product3/1
  Constant9/1 -> Sum6/2
  Constant10/1 -> Sum7/2
  Step3/1 -> Product3/2
  Step2/1 -> Product2/2
  Constant12/1 -> Integrator5/1
  Sum6/1 -> Sin1/1
  Step1/1 -> Product1/2
  Product2/1 -> Mux/2
  Product3/1 -> Mux/3
  Mux/1 -> ABC/1

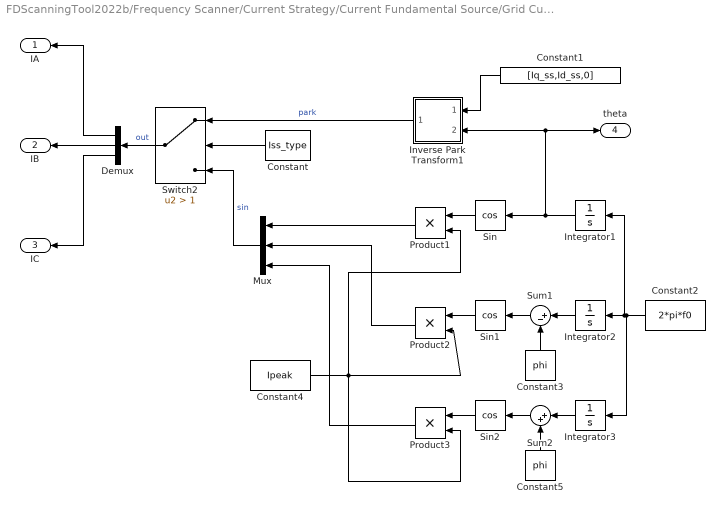
== system FDScanningTool2022b/Frequency Scanner/Current Strategy/Current Fundamental Source/Grid Currents1 ==
  Constant : Constant  Value=Iss_type
  Constant1 : Constant  Value=[Iq_ss,Id_ss,0]  SampleTime=delta_t
  Constant2 : Constant  Value=2*pi*f0
  Constant3 : Constant  Value=phi
  Constant4 : Constant  Value=Ipeak
  Constant5 : Constant  Value=phi
  Demux : Demux  Outputs=3
  Integrator1 : Integrator  UpperSaturationLimit=1E100  LowerSaturationLimit=-1E100
  Integrator2 : Integrator  UpperSaturationLimit=1E100  LowerSaturationLimit=-1E100
  Integrator3 : Integrator  UpperSaturationLimit=1E100  LowerSaturationLimit=-1E100
  Inverse Park Transform1 : Subsystem
  Mux : Mux  Inputs=3
  Product1 : Product
  Product2 : Product
  Product3 : Product
  Sin : Trigonometry  Operator=cos
  Sin1 : Trigonometry  Operator=cos
  Sin2 : Trigonometry  Operator=cos
  Sum1 : Sum  Inputs=|+-
  Sum2 : Sum  Inputs=|++
  Switch2 : Switch  Criteria=u2 > Threshold  Threshold=1  SaturateOnIntegerOverflow=off  InputSameDT=off
  IA : Outport
  IB : Outport  Port=2
  IC : Outport  Port=3
  theta : Outport  Port=4
  wires:
  Constant1/1 -> Inverse Park Transform1/1(qd0)
  Demux/1 -> IA/1
  Demux/2 -> IB/1
  Demux/3 -> IC/1
  Product3/1 -> Mux/3
  Product1/1 -> Mux/1
  Sum1/1 -> Sin1/1
  Integrator2/1 -> Sum1/1
  Constant5/1 -> Sum2/2
  Integrator3/1 -> Sum2/1
  Sin/1 -> Product1/1
  Sin2/1 -> Product3/1
  Sin1/1 -> Product2/1
  Sum2/1 -> Sin2/1
  Constant2/1 -> Integrator1/1, Integrator2/1, Integrator3/1
  Integrator1/1 -> theta/1, Inverse Park Transform1/2(theta), Sin/1
  Constant4/1 -> Product2/2, Product1/2, Product3/2
  Product2/1 -> Mux/2
  Constant3/1 -> Sum1/2
  Switch2/1 -> Demux/1  "out"
  Inverse Park Transform1/1(ABC) -> Switch2/1  "park"
  Mux/1 -> Switch2/3  "sin"
  Constant/1 -> Switch2/2

== system FDScanningTool2022b/Frequency Scanner/Current Strategy/pn0disturbance2/Fortescue Transformation ==
  note: This block buid a column vector with the inputs
      | M=[In1 In2 In3
      |       In1 In2 In3
      |       In1 In2 In3];
  ABC : Inport
  Constant{,3,46..47} (4 alike) : Constant  Value=0
  Constant1 : Constant  Value=(2/3)*pi
  Constant2 : Constant
  Constant43 : Constant
  Constant45 : Constant
  Math Function : Math
  Math Function1 : Math
  Matrix Concatenate : Concatenate  NumInputs=3  Mode=Multidimensional array  ConcatenateDimension=2
  Matrix Multiply : Product  Multiplication=Matrix(*)
  Multiply : Gain  Gain=1/3
  Mux1 : Mux  Inputs=3
  Mux2 : Mux  Inputs=3
  Mux3 : Mux  Inputs=3
  Real-Imag to Complex{,1..2,5} (4 alike) : RealImagToComplex
  Square : Math  Operator=square
  Square1 : Math  Operator=square
  0PN : Outport
  wires:
  Square/1 -> Mux1/3
  Math Function/1 -> Mux1/2, Square/1
  Real-Imag to Complex1/1 -> Mux3/1
  Square1/1 -> Mux3/2
  Multiply/1 -> Matrix Multiply/1
  Math Function1/1 -> Square1/1, Mux3/3
  Mux3/1 -> Matrix Concatenate/3
  Constant45/1 -> Real-Imag to Complex1/1
  Matrix Concatenate/1 -> Multiply/1
  Real-Imag to Complex2/1 -> Mux2/2, Mux2/1, Mux2/3
  Real-Imag to Complex5/1 -> Math Function1/1, Math Function/1
  ABC/1 -> Matrix Multiply/2
  Mux2/1 -> Matrix Concatenate/1
  Constant47/1 -> Real-Imag to Complex1/2
  Mux1/1 -> Matrix Concatenate/2
  Real-Imag to Complex/1 -> Mux1/1
  Constant46/1 -> Real-Imag to Complex/2
  Constant43/1 -> Real-Imag to Complex/1
  Matrix Multiply/1 -> 0PN/1
  Constant1/1 -> Real-Imag to Complex5/2
  Constant/1 -> Real-Imag to Complex5/1
  Constant2/1 -> Real-Imag to Complex2/1
  Constant3/1 -> Real-Imag to Complex2/2

== system FDScanningTool2022b/Frequency Scanner/Current Strategy/pn0disturbance2/Fortescue Transformation1 ==
  note: This block buid a column vector with the inputs
      | M=[In1 In2 In3
      |       In1 In2 In3
      |       In1 In2 In3];
  ABC : Inport
  Constant{,3,46..47} (4 alike) : Constant  Value=0
  Constant1 : Constant  Value=(2/3)*pi
  Constant2 : Constant
  Constant43 : Constant
  Constant45 : Constant
  Math Function : Math
  Math Function1 : Math
  Matrix Concatenate : Concatenate  NumInputs=3  Mode=Multidimensional array  ConcatenateDimension=2
  Matrix Multiply : Product  Multiplication=Matrix(*)
  Multiply : Gain  Gain=1/3
  Mux1 : Mux  Inputs=3
  Mux2 : Mux  Inputs=3
  Mux3 : Mux  Inputs=3
  Real-Imag to Complex{,1..2,5} (4 alike) : RealImagToComplex
  Square : Math  Operator=square
  Square1 : Math  Operator=square
  0PN : Outport
  wires:
  Square/1 -> Mux1/3
  Math Function/1 -> Mux1/2, Square/1
  Real-Imag to Complex1/1 -> Mux3/1
  Square1/1 -> Mux3/2
  Multiply/1 -> Matrix Multiply/1
  Math Function1/1 -> Square1/1, Mux3/3
  Mux3/1 -> Matrix Concatenate/3
  Constant45/1 -> Real-Imag to Complex1/1
  Matrix Concatenate/1 -> Multiply/1
  Real-Imag to Complex2/1 -> Mux2/2, Mux2/1, Mux2/3
  Real-Imag to Complex5/1 -> Math Function1/1, Math Function/1
  ABC/1 -> Matrix Multiply/2
  Mux2/1 -> Matrix Concatenate/1
  Constant47/1 -> Real-Imag to Complex1/2
  Mux1/1 -> Matrix Concatenate/2
  Real-Imag to Complex/1 -> Mux1/1
  Constant46/1 -> Real-Imag to Complex/2
  Constant43/1 -> Real-Imag to Complex/1
  Matrix Multiply/1 -> 0PN/1
  Constant1/1 -> Real-Imag to Complex5/2
  Constant/1 -> Real-Imag to Complex5/1
  Constant2/1 -> Real-Imag to Complex2/1
  Constant3/1 -> Real-Imag to Complex2/2

== system FDScanningTool2022b/Frequency Scanner/Current Strategy/pn0disturbance2/Multi-tone ==
  Clock : Clock
  Constant1 : Constant  Value=0
  From Workspace : FromWorkspace  VariableName=dist_value_0  SampleTime=delta_t  Interpolate=off  OutputAfterFinalValue=Holding final value
  From Workspace1 : FromWorkspace  VariableName=dist_value_p  SampleTime=delta_t  Interpolate=off  OutputAfterFinalValue=Holding final value
  From Workspace2 : FromWorkspace  VariableName=dist_value_n  SampleTime=delta_t  Interpolate=off  OutputAfterFinalValue=Holding final value
  Inverse Fortescue Transformation : Subsystem
  Mux : Mux  Inputs=3
  Switch1 : Switch  Criteria=u2 > Threshold  Threshold=dist_time  SaturateOnIntegerOverflow=off  InputSameDT=off
  Switch2 : Switch  Criteria=u2 > Threshold  Threshold=dist_time  SaturateOnIntegerOverflow=off  InputSameDT=off
  Switch3 : Switch  Criteria=u2 > Threshold  Threshold=dist_time  SaturateOnIntegerOverflow=off  InputSameDT=off
  ABC : Outport
  wires:
  Switch2/1 -> Mux/2
  From Workspace2/1 -> Switch3/1
  Constant1/1 -> Switch3/3, Switch2/3, Switch1/3
  From Workspace1/1 -> Switch2/1
  Switch3/1 -> Mux/3
  Clock/1 -> Switch1/2, Switch2/2, Switch3/2
  Switch1/1 -> Mux/1
  From Workspace/1 -> Switch1/1
  Mux/1 -> Inverse Fortescue Transformation/1(0PN)
  Inverse Fortescue Transformation/1(ABC) -> ABC/1

== system FDScanningTool2022b/Frequency Scanner/Current Strategy/pn0disturbance2/Single-tone ==
  Constant1 : Constant  Value=2*pi*fd  SampleTime=delta_t
  Constant1111 : Constant  Value=0
  Constant222 : Constant  Value=dist_value_p
  Constant49 : Constant  Value=dist_value_0
  Constant50 : Constant  Value=dist_value_n
  Disturbance activator : Step  Time=dist_time  SampleTime=delta_t
  Integrator3 : Integrator
  Inverse Fortescue Transformation : Subsystem
  Math Function3 : Math
  Math Function4 : Math
  Math Function5 : Math
  Multiply2 : Gain
  Multiply3 : Gain
  Multiply4 : Gain
  Mux1 : Mux  Inputs=3
  Product{,4..5,8} (4 alike) : Product
  Real-Imag to Complex2 : RealImagToComplex
  Real-Imag to Complex3 : RealImagToComplex
  Real-Imag to Complex4 : RealImagToComplex
  ABC : Outport
  wires:
  Real-Imag to Complex3/1 -> Multiply2/1
  Math Function3/1 -> Product5/2
  Real-Imag to Complex2/1 -> Multiply3/1
  Inverse Fortescue Transformation/1(ABC) -> Product/2
  Disturbance activator/1 -> Product/1
  Product8/1 -> Mux1/2
  Integrator3/1 -> Real-Imag to Complex2/2, Real-Imag to Complex3/2, Real-Imag to Complex4/2
  Product/1 -> ABC/1
  Multiply2/1 -> Math Function4/1
  Real-Imag to Complex4/1 -> Multiply4/1
  Constant222/1 -> Product8/2
  Math Function5/1 -> Product4/2
  Constant49/1 -> Product4/1
  Mux1/1 -> Inverse Fortescue Transformation/1(0PN)
  Multiply3/1 -> Math Function3/1
  Multiply4/1 -> Math Function5/1
  Constant1/1 -> Integrator3/1
  Product4/1 -> Mux1/1
  Math Function4/1 -> Product8/1
  Constant1111/1 -> Real-Imag to Complex4/1, Real-Imag to Complex3/1, Real-Imag to Complex2/1
  Product5/1 -> Mux1/3
  Constant50/1 -> Product5/1

== system FDScanningTool2022b/Frequency Scanner/Current Strategy/qd0disturbance2/Multi-tone ==
  In1 : Inport
  Clock1 : Clock
  Constant : Constant  Value=0
  From Workspace3 : FromWorkspace  VariableName=dist_value_q  SampleTime=delta_t  Interpolate=off  OutputAfterFinalValue=Holding final value
  From Workspace4 : FromWorkspace  VariableName=dist_value_d  SampleTime=delta_t  Interpolate=off  OutputAfterFinalValue=Holding final value
  Inverse Park Transform1 : Subsystem
  Mux3 : Mux  Inputs=3
  Switch : Switch  Criteria=u2 > Threshold  Threshold=dist_time  SaturateOnIntegerOverflow=off  InputSameDT=off
  Switch4 : Switch  Criteria=u2 > Threshold  Threshold=dist_time  SaturateOnIntegerOverflow=off  InputSameDT=off
  Vd : Constant  Value=0
  ABC : Outport
  wires:
  Inverse Park Transform1/1(ABC) -> ABC/1
  From Workspace3/1 -> Switch/1
  Clock1/1 -> Switch/2, Switch4/2
  Switch4/1 -> Mux3/2  "vd"
  Constant/1 -> Switch4/3, Switch/3
  Mux3/1 -> Inverse Park Transform1/1(qd0)
  Vd/1 -> Mux3/3
  From Workspace4/1 -> Switch4/1
  Switch/1 -> Mux3/1  "vq"
  In1/1 -> Inverse Park Transform1/2(theta)

== system FDScanningTool2022b/Frequency Scanner/Current Strategy/qd0disturbance2/Park Transform ==
  ABC : Inport
  wt : Inport  Port=2
  Constant : Constant  Value=1/2
  Constant1 : Constant  Value=1/2
  Constant2 : Constant  Value=1/2
  Constant3 : Constant  Value=(2*pi)/3
  Constant4 : Constant  Value=(2*pi)/3
  Cos : Trigonometry  Operator=cos
  Cos1 : Trigonometry  Operator=cos
  Cos2 : Trigonometry  Operator=cos
  Gain : Gain  Gain=2/3
  Matrix Concatenate : Concatenate  NumInputs=3  Mode=Multidimensional array  ConcatenateDimension=2
  Matrix Multiply : Product  Multiplication=Matrix(*)
  Mux : Mux  Inputs=3
  Mux1 : Mux  Inputs=3
  Mux2 : Mux  Inputs=3
  Sin : Trigonometry
  Sin1 : Trigonometry
  Sin2 : Trigonometry
  Sum : Sum  Inputs=|+-
  Sum1 : Sum  Inputs=|++
  qd0 : Outport
  wires:
  Sum/1 -> Sin1/1, Cos1/1
  Constant1/1 -> Mux1/3
  Sin2/1 -> Mux2/2
  Gain/1 -> Matrix Multiply/1
  Cos/1 -> Mux/1
  Constant3/1 -> Sum/2
  wt/1 -> Cos/1, Sin/1, Sum/1, Sum1/1
  Sum1/1 -> Sin2/1, Cos2/1
  Mux1/1 -> Matrix Concatenate/2
  Sin/1 -> Mux/2
  Constant4/1 -> Sum1/2
  Constant2/1 -> Mux2/3
  Mux2/1 -> Matrix Concatenate/3
  Cos2/1 -> Mux2/1
  Constant/1 -> Mux/3
  Matrix Concatenate/1 -> Gain/1
  Cos1/1 -> Mux1/1
  Sin1/1 -> Mux1/2
  Mux/1 -> Matrix Concatenate/1
  ABC/1 -> Matrix Multiply/2
  Matrix Multiply/1 -> qd0/1

== system FDScanningTool2022b/Frequency Scanner/Current Strategy/qd0disturbance2/Park Transform1 ==
  ABC : Inport
  wt : Inport  Port=2
  Constant : Constant  Value=1/2
  Constant1 : Constant  Value=1/2
  Constant2 : Constant  Value=1/2
  Constant3 : Constant  Value=(2*pi)/3
  Constant4 : Constant  Value=(2*pi)/3
  Cos : Trigonometry  Operator=cos
  Cos1 : Trigonometry  Operator=cos
  Cos2 : Trigonometry  Operator=cos
  Gain : Gain  Gain=2/3
  Matrix Concatenate : Concatenate  NumInputs=3  Mode=Multidimensional array  ConcatenateDimension=2
  Matrix Multiply : Product  Multiplication=Matrix(*)
  Mux : Mux  Inputs=3
  Mux1 : Mux  Inputs=3
  Mux2 : Mux  Inputs=3
  Sin : Trigonometry
  Sin1 : Trigonometry
  Sin2 : Trigonometry
  Sum : Sum  Inputs=|+-
  Sum1 : Sum  Inputs=|++
  qd0 : Outport
  wires:
  Sum/1 -> Sin1/1, Cos1/1
  Constant1/1 -> Mux1/3
  Sin2/1 -> Mux2/2
  Gain/1 -> Matrix Multiply/1
  Cos/1 -> Mux/1
  Constant3/1 -> Sum/2
  wt/1 -> Cos/1, Sin/1, Sum/1, Sum1/1
  Sum1/1 -> Sin2/1, Cos2/1
  Mux1/1 -> Matrix Concatenate/2
  Sin/1 -> Mux/2
  Constant4/1 -> Sum1/2
  Constant2/1 -> Mux2/3
  Mux2/1 -> Matrix Concatenate/3
  Cos2/1 -> Mux2/1
  Constant/1 -> Mux/3
  Matrix Concatenate/1 -> Gain/1
  Cos1/1 -> Mux1/1
  Sin1/1 -> Mux1/2
  Mux/1 -> Matrix Concatenate/1
  ABC/1 -> Matrix Multiply/2
  Matrix Multiply/1 -> qd0/1

== system FDScanningTool2022b/Frequency Scanner/Current Strategy/qd0disturbance2/Single-tone ==
  note: qd disturbance
  In1 : Inport
  Constant18 : Constant  Value=dist_value_d
  Constant19 : Constant  Value=2*pi*fd
  Constant21 : Constant  Value=dist_value_q
  Cos : Trigonometry  Operator=cos
  Cos1 : Trigonometry  Operator=cos
  Disturbance activator : Step  Time=dist_time  Before=0.0  After=1.0  SampleTime=delta_t
  Integrator : Integrator
  Inverse Park Transform : Subsystem
  Mux23 : Mux  Inputs=3
  Product : Product
  Product4 : Product
  Product5 : Product
  V0 : Constant  Value=0
  ABC : Outport
  wires:
  Product/1 -> ABC/1
  Cos1/1 -> Product5/1
  Product4/1 -> Mux23/1
  Constant21/1 -> Product4/1
  Product5/1 -> Mux23/2
  Integrator/1 -> Cos/1, Cos1/1
  Cos/1 -> Product4/2
  Disturbance activator/1 -> Product/1
  Inverse Park Transform/1(ABC) -> Product/2
  Mux23/1 -> Inverse Park Transform/1(qd0)
  In1/1 -> Inverse Park Transform/2(theta)
  Constant18/1 -> Product5/2
  Constant19/1 -> Integrator/1
  V0/1 -> Mux23/3

== system FDScanningTool2022b/Frequency Scanner/Voltage Strategy/ABCdisturbance/Multi-tone ==
  Clock : Clock
  Constant1 : Constant  Value=0
  From Workspace : FromWorkspace  VariableName=dist_value_a  SampleTime=delta_t  Interpolate=off  OutputAfterFinalValue=Holding final value
  From Workspace1 : FromWorkspace  VariableName=dist_value_b  SampleTime=delta_t  Interpolate=off  OutputAfterFinalValue=Holding final value
  From Workspace2 : FromWorkspace  VariableName=dist_value_c  SampleTime=delta_t  Interpolate=off  OutputAfterFinalValue=Holding final value
  Mux : Mux  Inputs=3
  Switch1 : Switch  Criteria=u2 > Threshold  Threshold=dist_time  SaturateOnIntegerOverflow=off  InputSameDT=off
  Switch2 : Switch  Criteria=u2 > Threshold  Threshold=dist_time  SaturateOnIntegerOverflow=off  InputSameDT=off
  Switch3 : Switch  Criteria=u2 > Threshold  Threshold=dist_time  SaturateOnIntegerOverflow=off  InputSameDT=off
  ABC : Outport
  wires:
  Switch2/1 -> Mux/2
  From Workspace2/1 -> Switch3/1
  Constant1/1 -> Switch3/3, Switch2/3, Switch1/3
  From Workspace1/1 -> Switch2/1
  Switch3/1 -> Mux/3
  Clock/1 -> Switch1/2, Switch2/2, Switch3/2
  Switch1/1 -> Mux/1
  From Workspace/1 -> Switch1/1
  Mux/1 -> ABC/1

== system FDScanningTool2022b/Frequency Scanner/Voltage Strategy/ABCdisturbance/Single-tone ==
  note: ABC perturbance
  Constant10 : Constant  Value=phi
  Constant12 : Constant  Value=2*pi*fd  SampleTime=delta_t
  Constant9 : Constant  Value=phi
  Integrator5 : Integrator  UpperSaturationLimit=1E100  LowerSaturationLimit=-1E100
  Mux : Mux  Inputs=3
  Product1 : Product
  Product2 : Product
  Product3 : Product
  Sin : Trigonometry  Operator=cos
  Sin1 : Trigonometry  Operator=cos
  Sin2 : Trigonometry  Operator=cos
  Step1 : Step  Time=dist_time  After=dist_value_a  SampleTime=delta_t
  Step2 : Step  Time=dist_time  After=dist_value_b  SampleTime=delta_t
  Step3 : Step  Time=dist_time  After=dist_value_c  SampleTime=delta_t
  Sum6 : Sum  Inputs=|+-
  Sum7 : Sum  Inputs=|++
  ABC : Outport
  wires:
  Sin/1 -> Product1/1
  Sum7/1 -> Sin2/1
  Product1/1 -> Mux/1
  Integrator5/1 -> Sum7/1, Sin/1, Sum6/1
  Sin1/1 -> Product2/1
  Sin2/1 -> Product3/1
  Constant9/1 -> Sum6/2
  Constant10/1 -> Sum7/2
  Step3/1 -> Product3/2
  Step2/1 -> Product2/2
  Constant12/1 -> Integrator5/1
  Sum6/1 -> Sin1/1
  Step1/1 -> Product1/2
  Product2/1 -> Mux/2
  Product3/1 -> Mux/3
  Mux/1 -> ABC/1
